simulink model "PI_MPC_PMSM"  (R2018b)
settings: Solver=ode23s  StartTime=0.0  StopTime=0.9  FixedStep=Ts  EnableMultiTasking=on
InitFcn:
  | Ts = 10e-6;
  | 
  | R = 0.958;
  | Ld = 5.25e-3;
  | Lq = 12e-3;
  | Pn = 4;
  | flux = 0.1827;
undefined symbols (not defined in the file): DiscIntNeverNeededParam
libraries: powerlib x7, powerlib_extras x3, simulink x2
settings Model: Creator=SUN  LastModifiedBy=Baize
settings SolverCC: ZeroCrossControl=DisableAll
settings DataIOCC: LimitDataPoints=on  SaveFormat=Array  SignalLoggingSaveFormat=ModelDataLogs
settings OptimizationCC: ExpressionDepthLimit=2147483647  InitFltsAndDblsToZero=on  LifeSpan=inf
settings DebuggingCC: UnderspecifiedInitializationDetection=Classic  MergeDetectMultiDrivingBlocksExec=none  SolverPrmCheckMsg=warning  FcnCallInpInsideContextMsg=warning  StateNameClashWarn=warning  SFUnexpectedBacktrackingDiag=warning  SFNoUnconditionalDefaultTransitionDiag=warning  SFExecutionAtInitializationDiag=none
settings HardwareCC: ProdBitPerPointer=32  ProdBitPerSizeT=32  ProdBitPerPtrDiffT=32  ProdLargestAtomicFloat=None  ProdIntDivRoundTo=Undefined  ProdEndianess=Unspecified  ProdWordSize=32  ProdHWDeviceType=32-bit Generic
settings ModelReferenceCC: PropagateSignalLabelsOutOfModel=off
settings SFSimCC: SimUseLocalCustomCode=off
settings RTWCC: RTWUseLocalCustomCode=off
settings CodeAppCC: StateflowObjectComments=on
settings GRTTargetCC: TargetLangStandard=C89/C90 (ANSI)  CombineOutputUpdateFcns=off  GRTInterface=on
settings ConfigComp: CovMetricSettings=dw  CovSaveCumulativeToWorkspaceVar=on  CovSaveSingleToWorkspaceVar=on  CovExternalEMLEnable=off  CovSFcnEnable=off
settings SimscapeCC: SimscapeNormalizeSystem=off

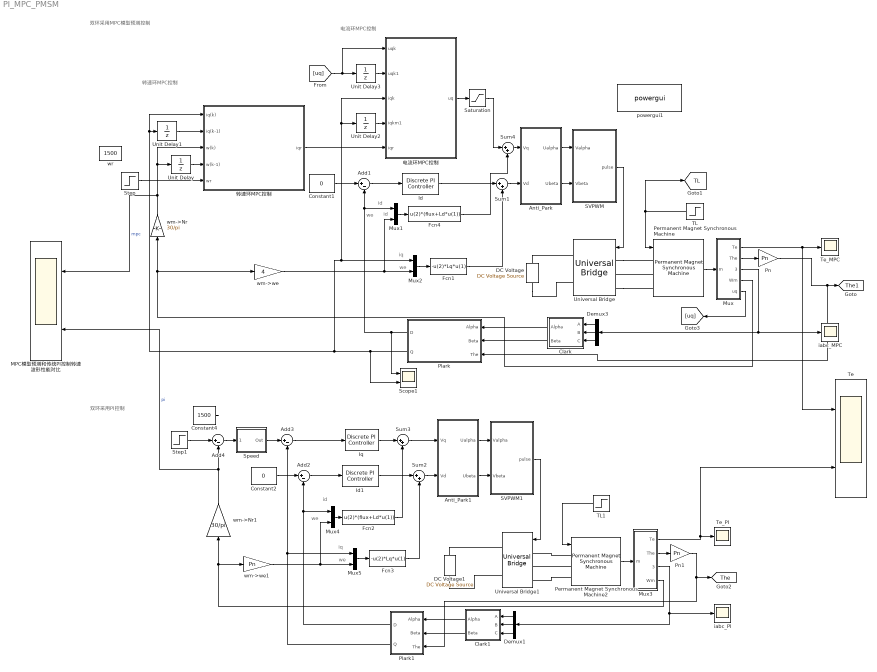
== system PI_MPC_PMSM ==
  note: 电流环MPC控制
  note: 转速环MPC控制
  note: 双环采用PI控制
  note: 双环采用MPC模型预测控制
  note: iq
  note: we
  note: id
  note: id
  note: iq
  note: we
  note: we
  note: we
  note: id
  Add{1..4} (4 alike) : Sum  Inputs=|+-
  Anti_Park : Subsystem
  Anti_Park1 : Subsystem
  Clark : Subsystem
  Clark1 : Subsystem
  Constant1 : Constant  Value=0
  Constant2 : Constant  Value=0
  Constant4 : Constant  Value=1500
  DC Voltage : powerlib/Electrical Sources/DC Voltage Source  Amplitude=540  Measurements=None
  DC Voltage1 : powerlib/Electrical Sources/DC Voltage Source  Amplitude=540  Measurements=None
  Demux1 : Demux  Outputs=3
  Demux3 : Demux  Outputs=3
  Fcn1 : Fcn  Expr=-u(2)*Lq*u(1)
  Fcn2 : Fcn  Expr=u(2)*(flux+Ld*u(1))
  Fcn3 : Fcn  Expr=-u(2)*Lq*u(1)
  Fcn4 : Fcn  Expr=u(2)*(flux+Ld*u(1))
  Id : powerlib_extras/Discrete  Control Blocks/Discrete PI Controller  Kp=Ld*1100  Ki=R*1100  Par_Limits=[311*0.9*sqrt(1/3) -311*0.9*sqrt(1/3)]  Init=0  Ts=Ts
  Id1 : powerlib_extras/Discrete  Control Blocks/Discrete PI Controller  Kp=Ld*1100  Ki=R*1100  Par_Limits=[311*0.9*sqrt(1/3) -311*0.9*sqrt(1/3)]  Init=0  Ts=Ts
  Iq : powerlib_extras/Discrete  Control Blocks/Discrete PI Controller  Kp=Lq*1100  Ki=R*1100  Par_Limits=[311*0.9*sqrt(1/3) -311*0.9*sqrt(1/3)]  Init=0  Ts=Ts
  MPC模型预测和传统PI控制转速波形性能对比 : Scope  NumInputPorts=2
  Mux : Subsystem
  Mux{1..2,4..5} (4 alike) : Mux  Inputs=2
  Mux3 : Subsystem
  Permanent Magnet Synchronous Machine : powerlib/Machines/Permanent Magnet Synchronous Machine  NbPhases=3  FluxDistribution=Sinusoidal  RotorType=Salient-pole  MechanicalLoad=Torque Tm  PresetModel=No  ShowDetailedParameters=on  MeasurementBus=off  Resistance=0.994  Inductance=8.5e-3  dqInductances=[6.3e-3,9e-3]  La=0.000395  MachineConstant=Flux linkage established by magnets (V.s)  Flux=0.3163  VoltageCst=229.4819  TorqueCst=1.8978  Flat=120  Mechanical=[0.014 0.009 4 0]  PolePairs=4  InitialConditions=[0,0,0,0]  InitialConditions5ph=[0 0 0 0 0 0]  TsPowergui=0  TsBlock=-1  RefAngle=Aligned with phase A axis (original Park)
      settings: SourceProductName=Simscape Power Systems
  Permanent Magnet Synchronous Machine2 : powerlib/Machines/Permanent Magnet Synchronous Machine  NbPhases=3  FluxDistribution=Sinusoidal  RotorType=Salient-pole  MechanicalLoad=Torque Tm  PresetModel=No  ShowDetailedParameters=on  MeasurementBus=off  Resistance=0.994  Inductance=8.5e-3  dqInductances=[6.3e-3,9e-3]  La=0.000395  MachineConstant=Flux linkage established by magnets (V.s)  Flux=0.3163  VoltageCst=229.4819  TorqueCst=1.8978  Flat=120  Mechanical=[0.014 0.009 4 0]  PolePairs=4  InitialConditions=[0,0,0,0]  InitialConditions5ph=[0 0 0 0 0 0]  TsPowergui=0  TsBlock=-1  RefAngle=Aligned with phase A axis (original Park)
      settings: SourceProductName=Simscape Power Systems
  Plark : Subsystem
  Plark1 : Subsystem
  Pn : Gain  Gain=Pn
  Pn1 : Gain  Gain=Pn
  SVPWM : Subsystem
  SVPWM1 : Subsystem
  Saturation : Saturate  UpperLimit=180  LowerLimit=-180
  Scope1 : Scope  NumInputPorts=2
  Speed : Subsystem  AncestorBlock=|  DialogController=POWERSYS.PowerSysDialog  mask(Discrete PI Controller){Kpw=0.14, Kiw=0.14*50, Ba=0.013, Par_Limits=[30 -30], Init=0, Ts=Ts}
      | powerlib_extras/Discrete 
      | Control Blocks/Discrete
      | PI Controller
      mask prompts: Kpw "Proportional gain (Kp):"; Kiw "Integral gain (Ki):"; Ba "feedback gain (Ba)"; Par_Limits "Output limits: [ Upper   Lower ]"; Init "Output initial value:"; Ts "Sample time:"
      mask help: This block implements a discrete PI controller.
      mask init:
      | UpperLimit=Par_Limits(1);
      | LowerLimit=Par_Limits(2);
      | power_initmask();
      mask Help: This block is part of a subset of blocks in the Extras library that does not have documentation associated with it, other than the block mask description.
      mask Display: disp('PI');
  Step : Step  Time=0.6  Before=1500  After=1300  SampleTime=0
  Step1 : Step  Time=0.6  Before=1500  After=1300  SampleTime=0
  Sum{1..4} (4 alike) : Sum  Inputs=|++
  TL : Step  Time=0.3  After=5  SampleTime=0
  TL1 : Step  Time=0.3  After=5  SampleTime=0
  Te : Scope  NumInputPorts=2
  Te_MPC : Scope
  Te_PI : Scope
  Unit Delay{,1..3} (4 alike) : UnitDelay  SampleTime=-1
  Universal Bridge : powerlib/Power Electronics/Universal Bridge  Arms=3  SnubberResistance=1e5  SnubberCapacitance=inf  Device=IGBT / Diodes  Ron=1e-3  Lon=0  ForwardVoltages="[  0  0  ]"  ForwardVoltage=0  GTOparameters=[ 10e-6 , 20e-6 ]  IGBTparameters=[ 1e-6 , 2e-6 ]  Measurements=None  Measurements_2=None  converterType=Rectifier
  Universal Bridge1 : powerlib/Power Electronics/Universal Bridge  Arms=3  SnubberResistance=1e5  SnubberCapacitance=inf  Device=IGBT / Diodes  Ron=1e-3  Lon=0  ForwardVoltages="[  0  0  ]"  ForwardVoltage=0  GTOparameters=[ 10e-6 , 20e-6 ]  IGBTparameters=[ 1e-6 , 2e-6 ]  Measurements=None  Measurements_2=None  converterType=Rectifier
  iabc_MPC : Scope
  iabc_PI : Scope
  powergui1 : powerlib/powergui  Priority=1  SimulationMode=Discrete  SampleTime=1e-6  frequency=60  Iterations=50  frequencyindice=0  Pbase=100e6  ErrMax=1e-4  UnitsV=kV  UnitsW=MW  buscounter=0  FunctionMessages=off  echomessages=off  EnableUseOfTLC=off  CurrentSourceSwitches=off  DisableSnubberDevices=off  DisableRonSwitches=off  DisableVfSwitches=off  DisplayEquations=off  SolverType=Tustin  Interpol=off  ExternalGateDelay=off  methode=off  Ts=10  x0status=blocks  SPID=off  SwTol=0  HookPort=off  RestoreLinks=warning  ResistiveCurrentMeasurement=off  Frange=[0:2:500]  Ylog=off  Xlog=on  ShowGrid=off  save=off  variable=ZData  structure=0  ZoomFFT=off  StartTime=0.0  cycles=1  DisplayStyle=1  fundamental=60  FreqAxis=off  MaxFrequency=1000  frequencyindicesteady=1  RmsSteady=1  display=off
  wm->Nr : Gain  Gain=30/pi
  wm->Nr1 : Gain  Gain=30/pi
  wm->we : Gain  Gain=4
  wm->we1 : Gain  Gain=Pn
  wr : Constant  Value=1500
  电流环MPC控制 : MATLAB Function  TreatAsAtomicUnit=on
  转速环MPC控制 : Subsystem
  tag scope: TL=global, The1=global, The=global
  wires:
  Permanent Magnet Synchronous Machine/1 -> Mux/1(m)
  Fcn1/1 -> Sum1/2
  Constant1/1 -> Add1/1
  Add1/1 -> Id/1
  wm->Nr/1 -> MPC模型预测和传统PI控制转速波形性能对比/1, 转速环MPC控制/3(w(k)), Unit Delay/1  "mpc"
  Id/1 -> Sum1/1
  Mux2/1 -> Fcn1/1
  Sum1/1 -> Anti_Park/2(Vd)
  Mux/1(Te) -> Te_MPC/1, Te/1
  Mux/2(The) -> Pn/1
  Pn/1 -> Plark/3(The), [The1]
  SVPWM/1(pulse) -> Universal Bridge/1
  Mux/4(Wm) -> wm->we/1, wm->Nr/1
  Mux/3(Iabc) -> iabc_MPC/1, Demux3/1
  Anti_Park/1(Ualpha) -> SVPWM/1(Valpha)
  Anti_Park/2(Ubeta) -> SVPWM/2(Vbeta)
  Clark/1(Alpha) -> Plark/1(Alpha)
  Demux3/1 -> Clark/1(A)
  Demux3/2 -> Clark/2(B)
  Demux3/3 -> Clark/3(C)
  Clark/2(Beta) -> Plark/2(Beta)
  TL/1 -> [TL], Permanent Magnet Synchronous Machine/1
  Unit Delay/1 -> 转速环MPC控制/4(w(k-1))
  Unit Delay1/1 -> 转速环MPC控制/2(iq(k-1))
  Step/1 -> 转速环MPC控制/5(wr)
  Add3/1 -> Iq/1
  Plark1/2(Q) -> Mux5/1, Add3/2
  Demux1/3 -> Clark1/3(C)
  SVPWM1/1(pulse) -> Universal Bridge1/1
  Mux3/2(The) -> Pn1/1
  Constant2/1 -> Add2/1
  Mux3/1(Te) -> Te/2, Te_PI/1
  Mux3/3(Iabc) -> iabc_PI/1, Demux1/1
  Sum2/1 -> Anti_Park1/2(Vd)
  Demux1/2 -> Clark1/2(B)
  Iq/1 -> Sum3/1
  Mux3/4(Wm) -> wm->we1/1, wm->Nr1/1
  Mux4/1 -> Fcn2/1
  Anti_Park1/2(Ubeta) -> SVPWM1/2(Vbeta)
  Add2/1 -> Id1/1
  wm->we1/1 -> Mux5/2, Mux4/2
  Constant4/1 -> ?
  Fcn3/1 -> Sum2/2
  Add4/1 -> Speed/1(Error)
  Permanent Magnet Synchronous Machine2/1 -> Mux3/1(m)
  Clark1/2(Beta) -> Plark1/2(Beta)
  wm->Nr1/1 -> Add4/2, MPC模型预测和传统PI控制转速波形性能对比/2  "pi"
  Demux1/1 -> Clark1/1(A)
  Speed/1(Out) -> Add3/1
  Mux5/1 -> Fcn3/1
  Id1/1 -> Sum2/1
  Clark1/1(Alpha) -> Plark1/1(Alpha)
  Plark1/1(D) -> Mux4/1, Add2/2
  Anti_Park1/1(Ualpha) -> SVPWM1/1(Valpha)
  Sum3/1 -> Anti_Park1/1(Vq)
  TL1/1 -> Permanent Magnet Synchronous Machine2/1
  Pn1/1 -> Plark1/3(The), [The]
  Fcn2/1 -> Sum3/2
  Plark/1(D) -> Scope1/1, Add1/2, Mux1/1
  Fcn4/1 -> Sum4/2
  Mux1/1 -> Fcn4/1
  wm->we/1 -> Mux2/2, Mux1/2
  Sum4/1 -> Anti_Park/1(Vq)
  Mux/5(uq) -> [uq]
  [uq] -> 电流环MPC控制/1(uqk), Unit Delay3/1
  Saturation/1 -> Sum4/1
  Unit Delay3/1 -> 电流环MPC控制/2(uqk1)
  电流环MPC控制/1(uq) -> Saturation/1
  Unit Delay2/1 -> 电流环MPC控制/4(iqkm1)
  转速环MPC控制/1(iqr) -> 电流环MPC控制/5(iqr)
  Plark/2(Q) -> Scope1/2, 转速环MPC控制/1(iq(k)), Unit Delay1/1, Mux2/1, 电流环MPC控制/3(iqk), Unit Delay2/1
  Step1/1 -> Add4/1
  connections:
  Permanent Magnet Synchronous Machine/LConn2 -- Universal Bridge/LConn2
  DC Voltage/RConn1 -- Universal Bridge/RConn1
  DC Voltage/LConn1 -- Universal Bridge/RConn2
  Universal Bridge/LConn3 -- Permanent Magnet Synchronous Machine/LConn3
  Universal Bridge/LConn1 -- Permanent Magnet Synchronous Machine/LConn1
  Permanent Magnet Synchronous Machine2/LConn2 -- Universal Bridge1/LConn2
  Permanent Magnet Synchronous Machine2/LConn1 -- Universal Bridge1/LConn1
  Permanent Magnet Synchronous Machine2/LConn3 -- Universal Bridge1/LConn3
  DC Voltage1/RConn1 -- Universal Bridge1/RConn1
  DC Voltage1/LConn1 -- Universal Bridge1/RConn2

== system PI_MPC_PMSM/Anti_Park ==
  Vq : Inport
  Vd : Inport  Port=2
  Fcn : Fcn  Expr=cos(u[1])*u[2]-sin(u[1])*u[3]
  Fcn1 : Fcn  Expr=sin(u[1])*u[2]+cos(u[1])*u[3]
  Mux1 : Mux  Inputs=3
  Ualpha : Outport  VectorParamsAs1DForOutWhenUnconnected=on
  Ubeta : Outport  Port=2  VectorParamsAs1DForOutWhenUnconnected=on
  wires:
  Fcn1/1 -> Ubeta/1
  Fcn/1 -> Ualpha/1
  Mux1/1 -> Fcn/1, Fcn1/1
  Vd/1 -> Mux1/2
  Vq/1 -> Mux1/3
  [The1] -> Mux1/1

== system PI_MPC_PMSM/Anti_Park1 ==
  Vq : Inport
  Vd : Inport  Port=2
  Fcn : Fcn  Expr=cos(u[1])*u[2]-sin(u[1])*u[3]
  Fcn1 : Fcn  Expr=sin(u[1])*u[2]+cos(u[1])*u[3]
  Mux1 : Mux  Inputs=3
  Ualpha : Outport  VectorParamsAs1DForOutWhenUnconnected=on
  Ubeta : Outport  Port=2  VectorParamsAs1DForOutWhenUnconnected=on
  wires:
  Fcn1/1 -> Ubeta/1
  Fcn/1 -> Ualpha/1
  Mux1/1 -> Fcn/1, Fcn1/1
  Vd/1 -> Mux1/2
  Vq/1 -> Mux1/3
  [The] -> Mux1/1

== system PI_MPC_PMSM/Clark ==
  A : Inport
  B : Inport  Port=2
  C : Inport  Port=3
  Mux : Mux  Inputs=3
  alpha : Fcn  Expr=(u(1)-0.5*(u(2)+u(3)))*2/3
  beta : Fcn  Expr=sqrt(3)/2*(u(2)-u(3))*2/3
  Alpha : Outport  VectorParamsAs1DForOutWhenUnconnected=on
  Beta : Outport  Port=2  VectorParamsAs1DForOutWhenUnconnected=on
  wires:
  alpha/1 -> Alpha/1
  B/1 -> Mux/2
  C/1 -> Mux/3
  A/1 -> Mux/1
  Mux/1 -> beta/1, alpha/1
  beta/1 -> Beta/1

== system PI_MPC_PMSM/Clark1 ==
  A : Inport
  B : Inport  Port=2
  C : Inport  Port=3
  Mux : Mux  Inputs=3
  alpha : Fcn  Expr=(u(1)-0.5*(u(2)+u(3)))*2/3
  beta : Fcn  Expr=sqrt(3)/2*(u(2)-u(3))*2/3
  Alpha : Outport  VectorParamsAs1DForOutWhenUnconnected=on
  Beta : Outport  Port=2  VectorParamsAs1DForOutWhenUnconnected=on
  wires:
  alpha/1 -> Alpha/1
  B/1 -> Mux/2
  C/1 -> Mux/3
  A/1 -> Mux/1
  Mux/1 -> beta/1, alpha/1
  beta/1 -> Beta/1

== system PI_MPC_PMSM/Mux ==
  m : Inport
  Bus Selector : BusSelector  OutputSignals=Stator current is_a (A),Stator current is_b (A),Stator current is_c (A)
  Bus Selector1 : BusSelector  OutputSignals=Rotor speed wm (rad/s),Rotor angle thetam (rad),Electromagnetic torque Te (N*m),Stator voltage Vs_q (V)
  Mux : Mux  Inputs=3
  Te : Outport  VectorParamsAs1DForOutWhenUnconnected=on
  The : Outport  Port=2  VectorParamsAs1DForOutWhenUnconnected=on
  Iabc : Outport  Port=3  VectorParamsAs1DForOutWhenUnconnected=on
  Wm : Outport  Port=4  VectorParamsAs1DForOutWhenUnconnected=on
  uq : Outport  Port=5  VectorParamsAs1DForOutWhenUnconnected=on
  wires:
  Bus Selector1/1 -> Wm/1  "<Rotor speed wm (rad/s)>"
  Bus Selector1/2 -> The/1  "<Rotor angle thetam (rad)>"
  Bus Selector1/3 -> Te/1  "<Electromagnetic torque Te (N*m)>"
  m/1 -> Bus Selector/1, Bus Selector1/1
  Bus Selector/2 -> Mux/2  "<Stator current is_b (A)>"
  Bus Selector/3 -> Mux/3  "<Stator current is_c (A)>"
  Bus Selector/1 -> Mux/1  "<Stator current is_a (A)>"
  Mux/1 -> Iabc/1
  Bus Selector1/4 -> uq/1  "<Stator voltage Vs_q (V)>"

== system PI_MPC_PMSM/Mux3 ==
  m : Inport
  Bus Selector : BusSelector  OutputSignals=Stator current is_a (A),Stator current is_b (A),Stator current is_c (A)
  Bus Selector1 : BusSelector  OutputSignals=Rotor speed wm (rad/s),Rotor angle thetam (rad),Electromagnetic torque Te (N*m)
  Mux : Mux  Inputs=3
  Te : Outport  VectorParamsAs1DForOutWhenUnconnected=on
  The : Outport  Port=2  VectorParamsAs1DForOutWhenUnconnected=on
  Iabc : Outport  Port=3  VectorParamsAs1DForOutWhenUnconnected=on
  Wm : Outport  Port=4  VectorParamsAs1DForOutWhenUnconnected=on
  wires:
  Bus Selector1/1 -> Wm/1  "<Rotor speed wm (rad/s)>"
  Bus Selector1/2 -> The/1  "<Rotor angle thetam (rad)>"
  Bus Selector1/3 -> Te/1  "<Electromagnetic torque Te (N*m)>"
  m/1 -> Bus Selector/1, Bus Selector1/1
  Bus Selector/2 -> Mux/2  "<Stator current is_b (A)>"
  Bus Selector/3 -> Mux/3  "<Stator current is_c (A)>"
  Bus Selector/1 -> Mux/1  "<Stator current is_a (A)>"
  Mux/1 -> Iabc/1

== system PI_MPC_PMSM/Plark ==
  Alpha : Inport
  Beta : Inport  Port=2
  The : Inport  Port=3
  Mux : Mux  Inputs=3
  d : Fcn  Expr=u(1)*cos(u(3))+u(2)*sin(u(3))
  q : Fcn  Expr=-u(1)*sin(u(3))+u(2)*cos(u(3))
  D : Outport  VectorParamsAs1DForOutWhenUnconnected=on
  Q : Outport  Port=2  VectorParamsAs1DForOutWhenUnconnected=on
  wires:
  d/1 -> D/1
  Beta/1 -> Mux/2
  Alpha/1 -> Mux/1
  Mux/1 -> q/1, d/1
  q/1 -> Q/1
  The/1 -> Mux/3

== system PI_MPC_PMSM/Plark1 ==
  Alpha : Inport
  Beta : Inport  Port=2
  The : Inport  Port=3
  Mux : Mux  Inputs=3
  d : Fcn  Expr=u(1)*cos(u(3))+u(2)*sin(u(3))
  q : Fcn  Expr=-u(1)*sin(u(3))+u(2)*cos(u(3))
  D : Outport  VectorParamsAs1DForOutWhenUnconnected=on
  Q : Outport  Port=2  VectorParamsAs1DForOutWhenUnconnected=on
  wires:
  d/1 -> D/1
  Beta/1 -> Mux/2
  Alpha/1 -> Mux/1
  Mux/1 -> q/1, d/1
  q/1 -> Q/1
  The/1 -> Mux/3

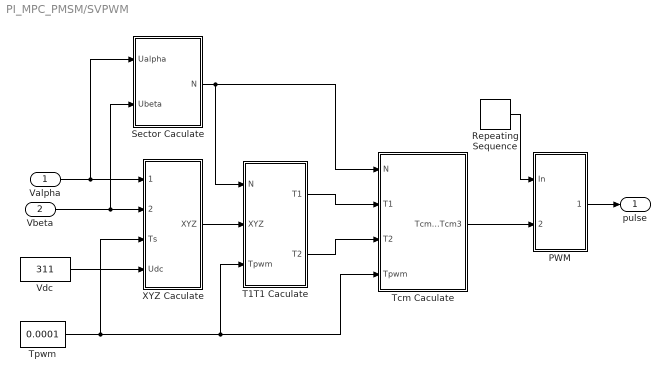
== system PI_MPC_PMSM/SVPWM ==
  Valpha : Inport
  Vbeta : Inport  Port=2
  PWM : Subsystem
  Repeating Sequence : simulink/Sources/Repeating Sequence  rep_seq_t=[0 0.00005 0.0001]  rep_seq_y=[0 0.00005 0]
  Sector Caculate : Subsystem
  T1T1 Caculate : Subsystem
  Tcm Caculate : Subsystem
  Tpwm : Constant  Value=0.0001
  Vdc : Constant  Value=311
  XYZ Caculate : Subsystem
  pulse : Outport  VectorParamsAs1DForOutWhenUnconnected=on
  wires:
  PWM/1(PWM) -> pulse/1
  Repeating Sequence/1 -> PWM/1(In)
  Vbeta/1 -> XYZ Caculate/2(Ubeta), Sector Caculate/2(Ubeta)
  T1T1 Caculate/1(T1) -> Tcm Caculate/2(T1)
  Valpha/1 -> XYZ Caculate/1(Ualpha), Sector Caculate/1(Ualpha)
  T1T1 Caculate/2(T2) -> Tcm Caculate/3(T2)
  Sector Caculate/1("N ") -> Tcm Caculate/1(N), T1T1 Caculate/1(N)
  XYZ Caculate/1(XYZ) -> T1T1 Caculate/2(XYZ)
  Tpwm/1 -> XYZ Caculate/3(Ts), Tcm Caculate/4(Tpwm), T1T1 Caculate/3(Tpwm)
  Vdc/1 -> XYZ Caculate/4(Udc)
  Tcm Caculate/1(Tcm1 Tcm2 Tcm3) -> PWM/2(Tcm123)

== system PI_MPC_PMSM/SVPWM1 ==
  Valpha : Inport
  Vbeta : Inport  Port=2
  PWM : Subsystem
  Repeating Sequence : simulink/Sources/Repeating Sequence  rep_seq_t=[0 0.00005 0.0001]  rep_seq_y=[0 0.00005 0]
  Sector Caculate : Subsystem
  T1T1 Caculate : Subsystem
  Tcm Caculate : Subsystem
  Tpwm : Constant  Value=0.0001
  Vdc : Constant  Value=311
  XYZ Caculate : Subsystem
  pulse : Outport  VectorParamsAs1DForOutWhenUnconnected=on
  wires:
  PWM/1(PWM) -> pulse/1
  Repeating Sequence/1 -> PWM/1(In)
  Vbeta/1 -> XYZ Caculate/2(Ubeta), Sector Caculate/2(Ubeta)
  T1T1 Caculate/1(T1) -> Tcm Caculate/2(T1)
  Valpha/1 -> XYZ Caculate/1(Ualpha), Sector Caculate/1(Ualpha)
  T1T1 Caculate/2(T2) -> Tcm Caculate/3(T2)
  Sector Caculate/1("N ") -> Tcm Caculate/1(N), T1T1 Caculate/1(N)
  XYZ Caculate/1(XYZ) -> T1T1 Caculate/2(XYZ)
  Tpwm/1 -> XYZ Caculate/3(Ts), Tcm Caculate/4(Tpwm), T1T1 Caculate/3(Tpwm)
  Vdc/1 -> XYZ Caculate/4(Udc)
  Tcm Caculate/1(Tcm1 Tcm2 Tcm3) -> PWM/2(Tcm123)

== system PI_MPC_PMSM/Speed ==
  note: Discrete PID Controller
  Error : Inport  SampleTime=Ts
  Discrete-Time Integrator : DiscreteIntegrator  InitialCondition=Init  SampleTime=Ts  LimitOutput=on  UpperSaturationLimit=UpperLimit  LowerSaturationLimit=LowerLimit  ICPrevOutput=DiscIntNeverNeededParam  ICPrevScaledInput=DiscIntNeverNeededParam
  Kp1 : Gain  Gain=Ba  SampleTime=Ts  SaturateOnIntegerOverflow=on  OutDataTypeStr=Inherit: Same as input  ParamDataTypeStr=Inherit: Same as input
  Kp4 : Gain  Gain=Kpw  SampleTime=Ts  SaturateOnIntegerOverflow=on  OutDataTypeStr=Inherit: Same as input  ParamDataTypeStr=Inherit: Same as input
  Kp5 : Gain  Gain=Kiw  SampleTime=Ts  SaturateOnIntegerOverflow=on  OutDataTypeStr=Inherit: Same as input  ParamDataTypeStr=Inherit: Same as input
  Saturation2 : Saturate  UpperLimit=UpperLimit  LowerLimit=LowerLimit  SampleTime=Ts
  Sum6 : Sum  Inputs=++-  SampleTime=Ts  SaturateOnIntegerOverflow=on  InputSameDT=on  OutDataTypeStr=Inherit: Same as first input
  Zero-Order Hold : ZeroOrderHold  SampleTime=Ts
  Out : Outport  SampleTime=Ts  InitialOutput=0  VectorParamsAs1DForOutWhenUnconnected=on
  wires:
  Error/1 -> Kp1/1, Kp5/1, Kp4/1
  Zero-Order Hold/1 -> Sum6/1
  Saturation2/1 -> Out/1
  Discrete-Time Integrator/1 -> Sum6/2
  Kp4/1 -> Zero-Order Hold/1
  Kp5/1 -> Discrete-Time Integrator/1
  Sum6/1 -> Saturation2/1
  Kp1/1 -> Sum6/3

== system PI_MPC_PMSM/转速环MPC控制 ==
  iq(k) : Inport
  iq(k-1) : Inport  Port=2
  w(k) : Inport  Port=3
  w(k-1) : Inport  Port=4
  wr : Inport  Port=5
  MATLAB Function : MATLAB Function  TreatAsAtomicUnit=on
  Saturation : Saturate  UpperLimit=30  LowerLimit=-30
  iqr : Outport  VectorParamsAs1DForOutWhenUnconnected=on
  wires:
  w(k-1)/1 -> MATLAB Function/4(wk1)
  iq(k-1)/1 -> MATLAB Function/2(iqk1)
  iq(k)/1 -> MATLAB Function/1(iqk)
  MATLAB Function/1(iq) -> Saturation/1
  w(k)/1 -> MATLAB Function/3(wk)
  wr/1 -> MATLAB Function/5(wr)
  Saturation/1 -> iqr/1
  [TL] -> MATLAB Function/6(TL)

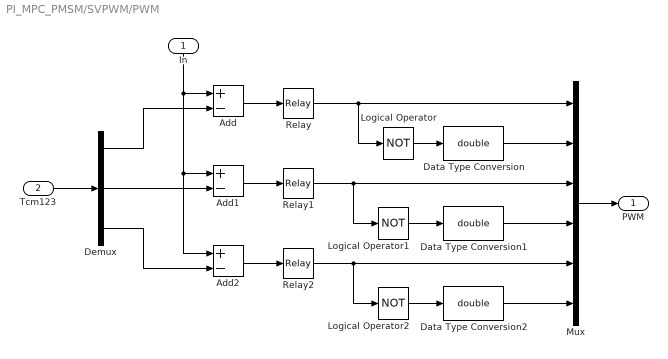
== system PI_MPC_PMSM/SVPWM/PWM ==
  In : Inport
  Tcm123 : Inport  Port=2
  Add : Sum  Inputs=+-
  Add1 : Sum  Inputs=+-
  Add2 : Sum  Inputs=+-
  Data Type Conversion : DataTypeConversion  OutDataTypeStr=double
  Data Type Conversion1 : DataTypeConversion  OutDataTypeStr=double
  Data Type Conversion2 : DataTypeConversion  OutDataTypeStr=double
  Demux : Demux  Outputs=3
  Logical Operator : Logic  Operator=NOT  AllPortsSameDT=off  OutDataTypeStr=boolean
  Logical Operator1 : Logic  Operator=NOT  AllPortsSameDT=off  OutDataTypeStr=boolean
  Logical Operator2 : Logic  Operator=NOT  AllPortsSameDT=off  OutDataTypeStr=boolean
  Mux : Mux  Inputs=6
  Relay : Relay  OffSwitchValue=-eps
  Relay1 : Relay  OffSwitchValue=-eps
  Relay2 : Relay  OffSwitchValue=-eps
  PWM : Outport  VectorParamsAs1DForOutWhenUnconnected=on
  wires:
  Demux/3 -> Add2/2
  Demux/2 -> Add1/2
  Demux/1 -> Add/2
  Relay2/1 -> Mux/5, Logical Operator2/1
  Relay1/1 -> Mux/3, Logical Operator1/1
  Relay/1 -> Logical Operator/1, Mux/1
  Mux/1 -> PWM/1
  Data Type Conversion/1 -> Mux/2
  Data Type Conversion1/1 -> Mux/4
  Data Type Conversion2/1 -> Mux/6
  Logical Operator2/1 -> Data Type Conversion2/1
  Logical Operator1/1 -> Data Type Conversion1/1
  Logical Operator/1 -> Data Type Conversion/1
  Add1/1 -> Relay1/1
  Add2/1 -> Relay2/1
  Add/1 -> Relay/1
  In/1 -> Add/1, Add2/1, Add1/1
  Tcm123/1 -> Demux/1

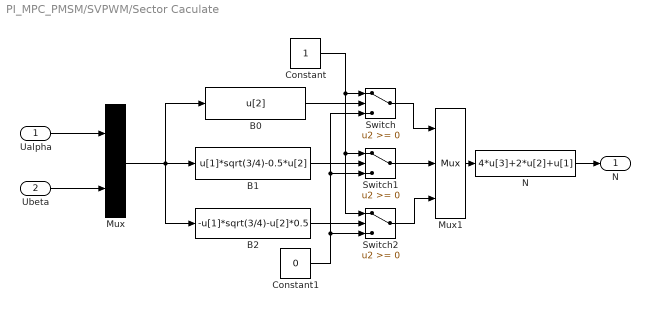
== system PI_MPC_PMSM/SVPWM/Sector Caculate ==
  Ualpha : Inport
  Ubeta : Inport  Port=2
  B0 : Fcn  Expr=u[2]
  B1 : Fcn  Expr=u[1]*sqrt(3/4)-0.5*u[2]
  B2 : Fcn  Expr=-u[1]*sqrt(3/4)-u[2]*0.5
  Constant : Constant
  Constant1 : Constant  Value=0
  Mux : Mux  Inputs=2
  Mux1 : Mux  Inputs=3
  N : Fcn  Expr=4*u[3]+2*u[2]+u[1]
  Switch : Switch
  Switch1 : Switch
  Switch2 : Switch
  "N " : Outport  VectorParamsAs1DForOutWhenUnconnected=on
  wires:
  Switch2/1 -> Mux1/3
  Switch/1 -> Mux1/1
  Ualpha/1 -> Mux/1
  Ubeta/1 -> Mux/2
  Mux/1 -> B2/1, B1/1, B0/1
  B0/1 -> Switch/2
  B1/1 -> Switch1/2
  B2/1 -> Switch2/2
  Constant/1 -> Switch/1, Switch2/1, Switch1/1
  Constant1/1 -> Switch/3, Switch1/3, Switch2/3
  Switch1/1 -> Mux1/2
  Mux1/1 -> N/1
  N/1 -> "N "/1

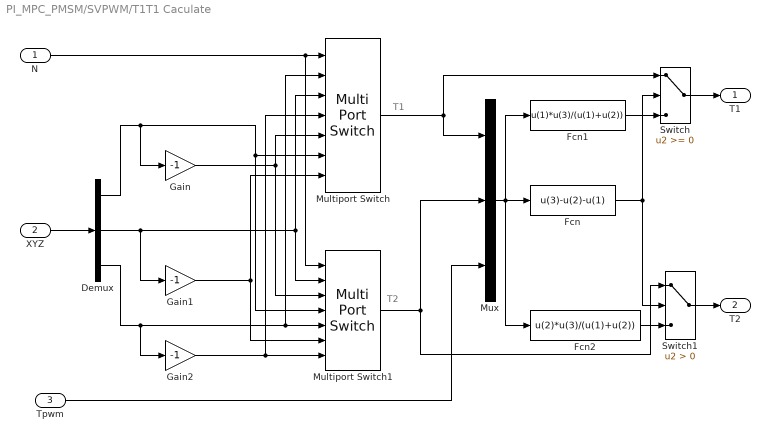
== system PI_MPC_PMSM/SVPWM/T1T1 Caculate ==
  note: T1
  note: T2
  N : Inport
  XYZ : Inport  Port=2
  Tpwm : Inport  Port=3
  Demux : Demux  Outputs=3
  Fcn : Fcn  Expr=u(3)-u(2)-u(1)
  Fcn1 : Fcn  Expr=u(1)*u(3)/(u(1)+u(2))
  Fcn2 : Fcn  Expr=u(2)*u(3)/(u(1)+u(2))
  Gain : Gain  Gain=-1
  Gain1 : Gain  Gain=-1
  Gain2 : Gain  Gain=-1
  Multiport Switch : MultiPortSwitch  Inputs=6
  Multiport Switch1 : MultiPortSwitch  Inputs=6
  Mux : Mux  Inputs=3
  Switch : Switch
  Switch1 : Switch  Criteria=u2 > Threshold
  T1 : Outport  VectorParamsAs1DForOutWhenUnconnected=on
  T2 : Outport  Port=2  VectorParamsAs1DForOutWhenUnconnected=on
  wires:
  Tpwm/1 -> Mux/3
  XYZ/1 -> Demux/1
  Switch1/1 -> T2/1
  Switch/1 -> T1/1
  Fcn2/1 -> Switch1/3
  Fcn1/1 -> Switch/3
  Fcn/1 -> Switch/2, Switch1/2
  Mux/1 -> Fcn1/1, Fcn/1, Fcn2/1
  Multiport Switch/1 -> Switch/1, Mux/1
  Multiport Switch1/1 -> Switch1/1, Mux/2
  N/1 -> Multiport Switch/1, Multiport Switch1/1
  Demux/2 -> Multiport Switch/3, Multiport Switch1/2, Gain1/1
  Demux/3 -> Multiport Switch1/5, Multiport Switch/2, Gain2/1
  Demux/1 -> Multiport Switch/6, Multiport Switch1/4, Gain/1
  Gain/1 -> Multiport Switch1/3, Multiport Switch/5
  Gain2/1 -> Multiport Switch/4, Multiport Switch1/7
  Gain1/1 -> Multiport Switch1/6, Multiport Switch/7

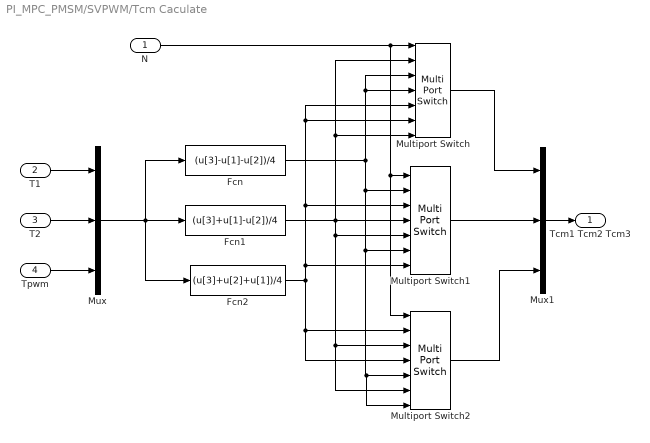
== system PI_MPC_PMSM/SVPWM/Tcm Caculate ==
  N : Inport
  T1 : Inport  Port=2
  T2 : Inport  Port=3
  Tpwm : Inport  Port=4
  Fcn : Fcn  Expr=(u[3]-u[1]-u[2])/4
  Fcn1 : Fcn  Expr=(u[3]+u[1]-u[2])/4
  Fcn2 : Fcn  Expr=(u[3]+u[2]+u[1])/4
  Multiport Switch : MultiPortSwitch  Inputs=6
  Multiport Switch1 : MultiPortSwitch  Inputs=6
  Multiport Switch2 : MultiPortSwitch  Inputs=6
  Mux : Mux  Inputs=3
  Mux1 : Mux  Inputs=3
  Tcm1 Tcm2 Tcm3 : Outport  VectorParamsAs1DForOutWhenUnconnected=on
  wires:
  Mux/1 -> Fcn2/1, Fcn/1, Fcn1/1
  Tpwm/1 -> Mux/3
  T2/1 -> Mux/2
  T1/1 -> Mux/1
  Multiport Switch2/1 -> Mux1/3
  Multiport Switch1/1 -> Mux1/2
  Multiport Switch/1 -> Mux1/1
  Mux1/1 -> Tcm1 Tcm2 Tcm3/1
  Fcn/1 -> Multiport Switch/3, Multiport Switch/4, Multiport Switch1/6, Multiport Switch2/5, Multiport Switch2/7, Multiport Switch1/2
  Fcn1/1 -> Multiport Switch1/5, Multiport Switch2/3, Multiport Switch2/6, Multiport Switch1/4, Multiport Switch/7, Multiport Switch/2
  Fcn2/1 -> Multiport Switch/5, Multiport Switch/6, Multiport Switch1/3, Multiport Switch1/7, Multiport Switch2/2, Multiport Switch2/4
  N/1 -> Multiport Switch2/1, Multiport Switch1/1, Multiport Switch/1

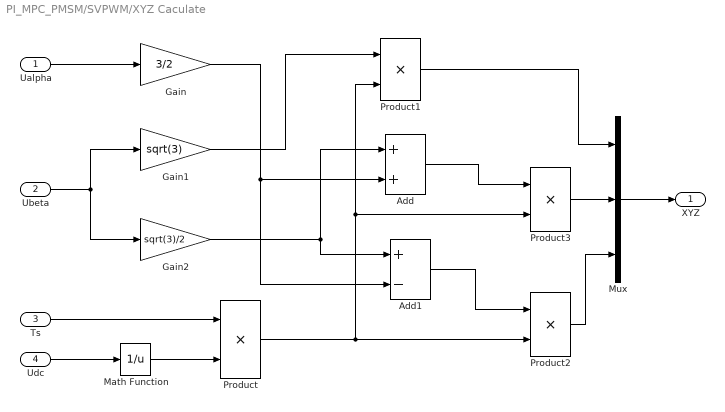
== system PI_MPC_PMSM/SVPWM/XYZ Caculate ==
  Ualpha : Inport
  Ubeta : Inport  Port=2
  Ts : Inport  Port=3
  Udc : Inport  Port=4
  Add : Sum
  Add1 : Sum  Inputs=+-
  Gain : Gain  Gain=3/2
  Gain1 : Gain  Gain=sqrt(3)
  Gain2 : Gain  Gain=sqrt(3)/2
  Math Function : Math  Operator=reciprocal  SaturateOnIntegerOverflow=on
  Mux : Mux  Inputs=3
  Product{,1..3} (4 alike) : Product  RndMeth=Zero
  XYZ : Outport  VectorParamsAs1DForOutWhenUnconnected=on
  wires:
  Mux/1 -> XYZ/1
  Product1/1 -> Mux/1
  Product3/1 -> Mux/2
  Product2/1 -> Mux/3
  Ualpha/1 -> Gain/1
  Ubeta/1 -> Gain2/1, Gain1/1
  Udc/1 -> Math Function/1
  Math Function/1 -> Product/2
  Ts/1 -> Product/1
  Gain1/1 -> Product1/1
  Product/1 -> Product2/2, Product1/2, Product3/2
  Gain/1 -> Add1/2, Add/2
  Gain2/1 -> Add/1, Add1/1
  Add1/1 -> Product2/1
  Add/1 -> Product3/1

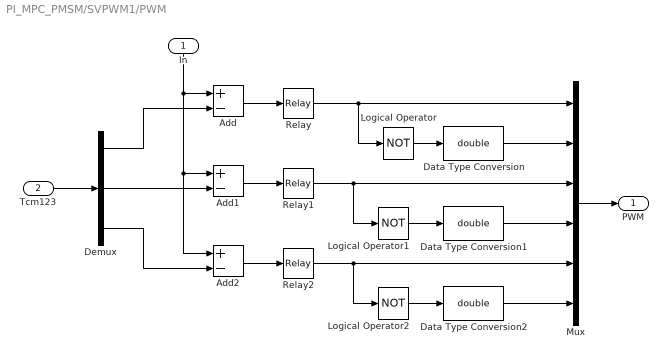
== system PI_MPC_PMSM/SVPWM1/PWM ==
  In : Inport
  Tcm123 : Inport  Port=2
  Add : Sum  Inputs=+-
  Add1 : Sum  Inputs=+-
  Add2 : Sum  Inputs=+-
  Data Type Conversion : DataTypeConversion  OutDataTypeStr=double
  Data Type Conversion1 : DataTypeConversion  OutDataTypeStr=double
  Data Type Conversion2 : DataTypeConversion  OutDataTypeStr=double
  Demux : Demux  Outputs=3
  Logical Operator : Logic  Operator=NOT  AllPortsSameDT=off  OutDataTypeStr=boolean
  Logical Operator1 : Logic  Operator=NOT  AllPortsSameDT=off  OutDataTypeStr=boolean
  Logical Operator2 : Logic  Operator=NOT  AllPortsSameDT=off  OutDataTypeStr=boolean
  Mux : Mux  Inputs=6
  Relay : Relay  OffSwitchValue=-eps
  Relay1 : Relay  OffSwitchValue=-eps
  Relay2 : Relay  OffSwitchValue=-eps
  PWM : Outport  VectorParamsAs1DForOutWhenUnconnected=on
  wires:
  Demux/3 -> Add2/2
  Demux/2 -> Add1/2
  Demux/1 -> Add/2
  Relay2/1 -> Mux/5, Logical Operator2/1
  Relay1/1 -> Mux/3, Logical Operator1/1
  Relay/1 -> Logical Operator/1, Mux/1
  Mux/1 -> PWM/1
  Data Type Conversion/1 -> Mux/2
  Data Type Conversion1/1 -> Mux/4
  Data Type Conversion2/1 -> Mux/6
  Logical Operator2/1 -> Data Type Conversion2/1
  Logical Operator1/1 -> Data Type Conversion1/1
  Logical Operator/1 -> Data Type Conversion/1
  Add1/1 -> Relay1/1
  Add2/1 -> Relay2/1
  Add/1 -> Relay/1
  In/1 -> Add/1, Add2/1, Add1/1
  Tcm123/1 -> Demux/1

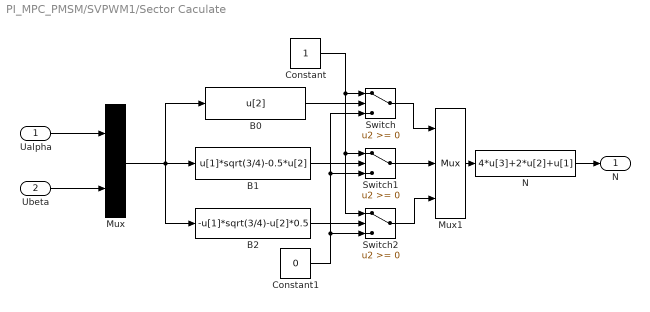
== system PI_MPC_PMSM/SVPWM1/Sector Caculate ==
  Ualpha : Inport
  Ubeta : Inport  Port=2
  B0 : Fcn  Expr=u[2]
  B1 : Fcn  Expr=u[1]*sqrt(3/4)-0.5*u[2]
  B2 : Fcn  Expr=-u[1]*sqrt(3/4)-u[2]*0.5
  Constant : Constant
  Constant1 : Constant  Value=0
  Mux : Mux  Inputs=2
  Mux1 : Mux  Inputs=3
  N : Fcn  Expr=4*u[3]+2*u[2]+u[1]
  Switch : Switch
  Switch1 : Switch
  Switch2 : Switch
  "N " : Outport  VectorParamsAs1DForOutWhenUnconnected=on
  wires:
  Switch2/1 -> Mux1/3
  Switch/1 -> Mux1/1
  Ualpha/1 -> Mux/1
  Ubeta/1 -> Mux/2
  Mux/1 -> B2/1, B1/1, B0/1
  B0/1 -> Switch/2
  B1/1 -> Switch1/2
  B2/1 -> Switch2/2
  Constant/1 -> Switch/1, Switch2/1, Switch1/1
  Constant1/1 -> Switch/3, Switch1/3, Switch2/3
  Switch1/1 -> Mux1/2
  Mux1/1 -> N/1
  N/1 -> "N "/1

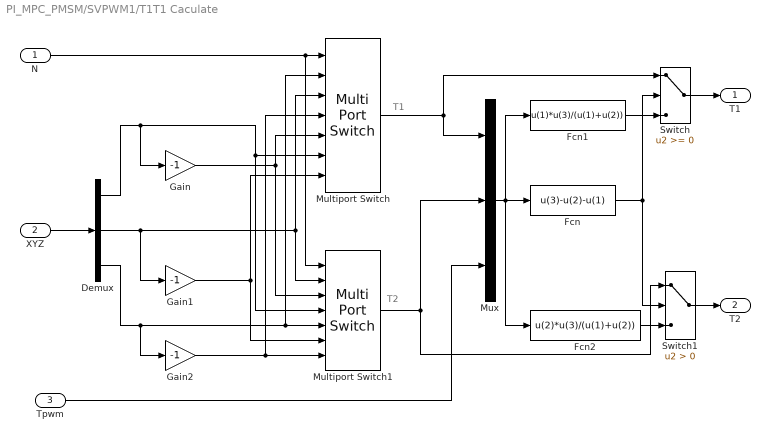
== system PI_MPC_PMSM/SVPWM1/T1T1 Caculate ==
  note: T1
  note: T2
  N : Inport
  XYZ : Inport  Port=2
  Tpwm : Inport  Port=3
  Demux : Demux  Outputs=3
  Fcn : Fcn  Expr=u(3)-u(2)-u(1)
  Fcn1 : Fcn  Expr=u(1)*u(3)/(u(1)+u(2))
  Fcn2 : Fcn  Expr=u(2)*u(3)/(u(1)+u(2))
  Gain : Gain  Gain=-1
  Gain1 : Gain  Gain=-1
  Gain2 : Gain  Gain=-1
  Multiport Switch : MultiPortSwitch  Inputs=6
  Multiport Switch1 : MultiPortSwitch  Inputs=6
  Mux : Mux  Inputs=3
  Switch : Switch
  Switch1 : Switch  Criteria=u2 > Threshold
  T1 : Outport  VectorParamsAs1DForOutWhenUnconnected=on
  T2 : Outport  Port=2  VectorParamsAs1DForOutWhenUnconnected=on
  wires:
  Tpwm/1 -> Mux/3
  XYZ/1 -> Demux/1
  Switch1/1 -> T2/1
  Switch/1 -> T1/1
  Fcn2/1 -> Switch1/3
  Fcn1/1 -> Switch/3
  Fcn/1 -> Switch/2, Switch1/2
  Mux/1 -> Fcn1/1, Fcn/1, Fcn2/1
  Multiport Switch/1 -> Switch/1, Mux/1
  Multiport Switch1/1 -> Switch1/1, Mux/2
  N/1 -> Multiport Switch/1, Multiport Switch1/1
  Demux/2 -> Multiport Switch/3, Multiport Switch1/2, Gain1/1
  Demux/3 -> Multiport Switch1/5, Multiport Switch/2, Gain2/1
  Demux/1 -> Multiport Switch/6, Multiport Switch1/4, Gain/1
  Gain/1 -> Multiport Switch1/3, Multiport Switch/5
  Gain2/1 -> Multiport Switch/4, Multiport Switch1/7
  Gain1/1 -> Multiport Switch1/6, Multiport Switch/7

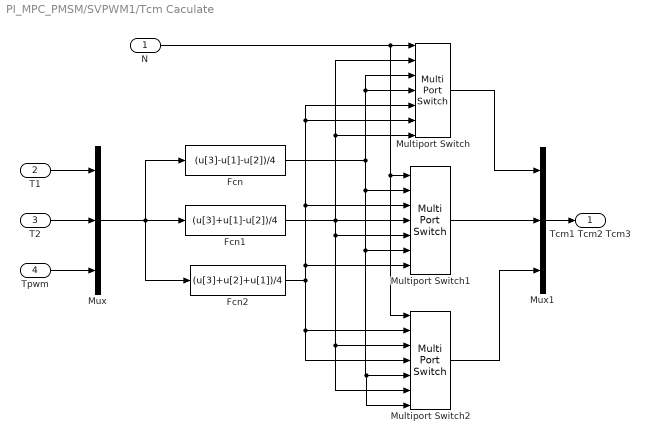
== system PI_MPC_PMSM/SVPWM1/Tcm Caculate ==
  N : Inport
  T1 : Inport  Port=2
  T2 : Inport  Port=3
  Tpwm : Inport  Port=4
  Fcn : Fcn  Expr=(u[3]-u[1]-u[2])/4
  Fcn1 : Fcn  Expr=(u[3]+u[1]-u[2])/4
  Fcn2 : Fcn  Expr=(u[3]+u[2]+u[1])/4
  Multiport Switch : MultiPortSwitch  Inputs=6
  Multiport Switch1 : MultiPortSwitch  Inputs=6
  Multiport Switch2 : MultiPortSwitch  Inputs=6
  Mux : Mux  Inputs=3
  Mux1 : Mux  Inputs=3
  Tcm1 Tcm2 Tcm3 : Outport  VectorParamsAs1DForOutWhenUnconnected=on
  wires:
  Mux/1 -> Fcn2/1, Fcn/1, Fcn1/1
  Tpwm/1 -> Mux/3
  T2/1 -> Mux/2
  T1/1 -> Mux/1
  Multiport Switch2/1 -> Mux1/3
  Multiport Switch1/1 -> Mux1/2
  Multiport Switch/1 -> Mux1/1
  Mux1/1 -> Tcm1 Tcm2 Tcm3/1
  Fcn/1 -> Multiport Switch/3, Multiport Switch/4, Multiport Switch1/6, Multiport Switch2/5, Multiport Switch2/7, Multiport Switch1/2
  Fcn1/1 -> Multiport Switch1/5, Multiport Switch2/3, Multiport Switch2/6, Multiport Switch1/4, Multiport Switch/7, Multiport Switch/2
  Fcn2/1 -> Multiport Switch/5, Multiport Switch/6, Multiport Switch1/3, Multiport Switch1/7, Multiport Switch2/2, Multiport Switch2/4
  N/1 -> Multiport Switch2/1, Multiport Switch1/1, Multiport Switch/1

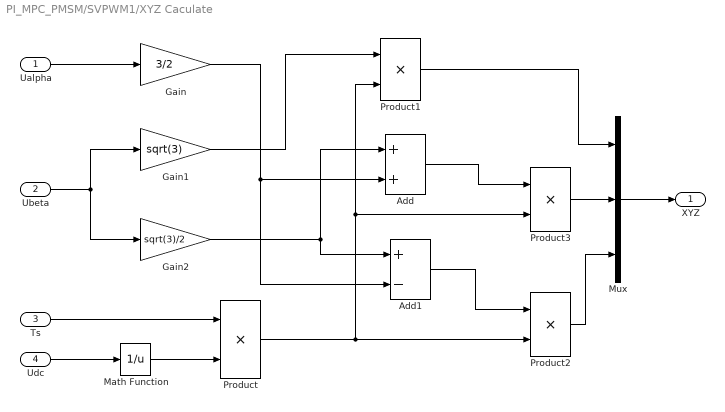
== system PI_MPC_PMSM/SVPWM1/XYZ Caculate ==
  Ualpha : Inport
  Ubeta : Inport  Port=2
  Ts : Inport  Port=3
  Udc : Inport  Port=4
  Add : Sum
  Add1 : Sum  Inputs=+-
  Gain : Gain  Gain=3/2
  Gain1 : Gain  Gain=sqrt(3)
  Gain2 : Gain  Gain=sqrt(3)/2
  Math Function : Math  Operator=reciprocal  SaturateOnIntegerOverflow=on
  Mux : Mux  Inputs=3
  Product{,1..3} (4 alike) : Product  RndMeth=Zero
  XYZ : Outport  VectorParamsAs1DForOutWhenUnconnected=on
  wires:
  Mux/1 -> XYZ/1
  Product1/1 -> Mux/1
  Product3/1 -> Mux/2
  Product2/1 -> Mux/3
  Ualpha/1 -> Gain/1
  Ubeta/1 -> Gain2/1, Gain1/1
  Udc/1 -> Math Function/1
  Math Function/1 -> Product/2
  Ts/1 -> Product/1
  Gain1/1 -> Product1/1
  Product/1 -> Product2/2, Product1/2, Product3/2
  Gain/1 -> Add1/2, Add/2
  Gain2/1 -> Add/1, Add1/1
  Add1/1 -> Product2/1
  Add/1 -> Product3/1

== matlab function PI_MPC_PMSM/电流环MPC控制 ==
  data: uqk input; uq output; uqk1 input; iqk input; iqkm1 input; iqr input
function uq = fcn(uqk,uqk1,iqk,iqkm1,iqr)
% q轴电流的模型预测控制：先基于电机q轴电压方程推导离散化电流预测模型，计算预测时域内仅由历史电流决定的电流预测值及电压对电流的影响系数；
% 通过对比实际预测电流与初步预测电流得到误差，校正电流参考值；
% 最后构建包含电流跟踪误差和控制量变化的目标函数，求解二次规划得到最优电压增量，输出下一时刻q轴电压控制量，实现电流精准跟踪。

% fcn - 永磁同步电机(q轴)电流预测控制核心计算函数
% 输入参数:
%   uqk    : 当前k时刻的q轴电压控制量 (V)
%   uqk1   : 上一时刻(k-1)的q轴电压控制量 (V)
%   iqk    : 当前k时刻的q轴电流反馈值 (A)
%   iqkm1  : 上一时刻(k-1)的q轴电流反馈值 (A)
%   iqr    : q轴电流参考值（电流环给定）(A)
% 输出参数:
%   uq     : 计算得到的下一时刻q轴电压控制量 (V)

%% 1. 定义电机及控制系统固定参数
ff=0.3163;               % 电机相关系数（未在计算中使用）
Rs=0.994;                % 定子相电阻 (Ω)
np=4;                    % 电机极对数（未在计算中使用）
Ts=1e-6;                 % 控制系统采样周期 (s)
Ld=6.3e-3;               % d轴电感 (H)
Lq=9e-3;                 % q轴电感 (H)
delta=0;                 % 误差校正系数（初始化为0，可根据系统调节）
N=4;                     % 模型预测控制(MPC)的预测时域长度
Nu=2;                    % 模型预测控制(MPC)的控制时域长度

%% 2. 推导离散化模型的系数
% 基于电机q轴电压方程：u_q = R_s*i_q + L_q*di_q/dt
% 离散化后得到：i_q(k+1) = C*i_q(k) + D*u_q(k)
C=1-Rs*Ts/Lq;            % 离散化模型系数C
D=Ts/Ld;                 % 离散化模型系数D（注：此处用Ld，需确认是否应为Lq）

%% 3. 初始化数组（存储预测时域内的中间变量）
Wiqm = zeros(N,1);       % 初始化：仅由历史电流决定的q轴电流预测值矩阵
Wuq = zeros(N,1);        % 初始化：电压控制量对电流预测值的影响系数矩阵
Wiqp = zeros(N,1);       % 初始化：综合后的q轴电流预测值矩阵
Iqr  = zeros(N,1);       % 初始化：经误差校正后的q轴电流参考值矩阵

%% 4. 计算预测时域内的电流预测系数矩阵
for i = 1:N
    Ci=0;
    Cj=0;
    Cn=0;
    
    % 计算系数Ci和Cj：用于Wiqm的计算
    for j = 0:N
       Ci = Ci+C^(j);          % 累加计算C的0到N次幂和
       Cj=Ci-1;                % Ci减去1，用于历史电流项的计算
    end
    
    % 计算系数Cn：用于Wuq的计算
    for j = 0:N-1
       Cn = Cn+(N-j)*C^(j);    % 带权重累加C的幂次和，权重为(N-j)
    end
    
    % 计算仅由历史电流决定的电流预测值
    Wiqm(i, 1) = Ci*iqk - Cj*iqkm1;
    % 计算电压控制量对电流预测的影响系数
    Wuq(i, 1) = Cn*D;
end

%% 5. 计算电压增量及初步电流预测值
dtuq0=uqk-uqk1;              % 计算当前时刻与上一时刻的q轴电压增量
Wiqp=Wiqm + Wuq.*dtuq0;      % 结合电压增量，计算初步的q轴电流预测值

%% 6. 误差计算与反馈校正
iqk1=C*iqk + D*uqk;          % 计算k+1时刻的q轴电流实际预测值
e=iqk1 - Wiqp(1,1);          % 计算"初步预测值"与"实际预测值"的误差

% 对预测时域内的电流参考值进行反馈校正（补偿模型误差）
for i = 1:N
    Iqr(i,1) = iqr + delta*e;    % 校正后的电流参考值 = 原始参考值 + 误差补偿项
end

%% 7. 模型预测控制的滚动优化求解
R=0.001*eye(Nu);             % 控制量增量的权重矩阵（惩罚过度的控制量变化）
Q=eye(N);                    % 电流跟踪误差的权重矩阵（强调跟踪精度）

% 求解二次规划问题，最小化目标函数 J = ||Iqr-Wiqm-Wuq*dtuq||_Q^2 + ||dtuq||_R^2
% 解析解：dtuq = inv(R^2 + Wuq'*Q*Wuq) * (Wuq'*Q*(Iqr-Wiqm))
dtuq=inv(R^(2)+Wuq'*Q*Wuq)*(Wuq'*Q*(Iqr-Wiqm));

% 取控制时域第一个控制量，计算最终输出的q轴电压
uq = dtuq(1,1) + uqk1;      % 最终控制量 = 电压增量 + 上一时刻电压值

end

== matlab function PI_MPC_PMSM/转速环MPC控制/MATLAB Function ==
  data: iqk input; iq output; iqk1 input; wk input; wk1 input; wr input; TL input
function iq = fcn(iqk,iqk1,wk,wk1,wr,TL)
% 转速环连续集模型预测控制：基于电机机械运动方程推导转速离散化模型，计算预测时域内仅由历史转速决定的转速预测值及 q 轴电流对转速的影响系数；
% 结合电流增量得到初步转速预测值，对比实际预测转速得到误差并校正转速参考值；
% 通过求解二次规划解析解得到最优q轴电流增量，输出最终q轴电流参考值，实现转速精准跟踪并抑制负载扰动。
%fcn - 永磁同步电机转速环模型预测控制(MPC)核心计算函数
% 输入参数:
%   iqk    : 当前k时刻的q轴电流反馈值 (A)，作为转速环的控制量
%   iqk1   : 上一时刻(k-1)的q轴电流反馈值 (A)
%   wk     : 当前k时刻的电机转速反馈值 (rad/s)
%   wk1    : 上一时刻(k-1)的电机转速反馈值 (rad/s)
%   wr     : 电机转速参考值（转速环给定）(rad/s)
%   TL     : 电机负载转矩扰动 (N·m)
% 输出参数:
%   iq     : 转速环输出的q轴电流参考值（送给电流环）(A)

%% 1. 定义电机及控制系统固定参数
ff=0.3163;               % 电机反电动势系数 (V/(rad/s))
Ts=1e-5;                 % 转速环采样周期 (s)
np=4;                    % 电机极对数
F=0.009;                 % 电机粘滞摩擦系数 (N·m/(rad/s))
J=0.014;                 % 电机转动惯量 (kg·m²)
delta=80;                % 转速预测误差校正系数（调节反馈校正强度）
N=4;                     % 模型预测控制(MPC)的预测时域长度
Nu=2;                    % 模型预测控制(MPC)的控制时域长度

%% 2. 推导转速离散化模型的核心系数
% 基于电机机械运动方程：J*dw/dt = T_e - T_L - F*w
% 电磁转矩 T_e = 1.5*np*ff*iq，代入后离散化得到：w(k+1) = A*w(k) + B*iq(k) - TL*Ts/J
A=1-F*Ts/J;              % 离散化模型系数A（转速自身衰减项）
B=1.5*np*ff*Ts/J;        % 离散化模型系数B（q轴电流对转速的影响项）

%% 3. 初始化数组（存储预测时域内的中间变量）
Wwm = zeros(N,1);        % 初始化：仅由历史转速决定的转速预测值矩阵
Wiq = zeros(N,1);        % 初始化：q轴电流对转速预测值的影响系数矩阵
Wwp = zeros(N,1);        % 初始化：综合后的转速预测值矩阵
Wr  = zeros(N,1);        % 初始化：经误差校正后的转速参考值矩阵
% N=4;  % 重复定义，注释掉（避免变量重复赋值）

%% 4. 计算预测时域内的转速预测系数矩阵
for i = 1:N
    Ai=0;
    Aj=0;
    An=0;
    
    % 计算系数Ai和Aj：用于Wwm（历史转速项）的计算
    for j = 0:N
       Ai = Ai+A^(j);          % 累加计算A的0到N次幂和
       Aj=Ai-1;                % Ai减去1，用于历史转速项的计算
    end
    
    % 计算系数An：用于Wiq（电流影响项）的计算
    for j = 0:N-1
       An = An+(N-j)*A^(j);    % 带权重累加A的幂次和，权重为(N-j)
    end
    
    % 计算仅由历史转速决定的转速预测值
    Wwm(i, 1) = Ai*wk - Aj*wk1;
    % 计算q轴电流对转速预测的影响系数
    Wiq(i, 1) = An*B;
end

%% 5. 计算电流增量及初步转速预测值
dtiq0=iqk-iqk1;              % 计算当前时刻与上一时刻的q轴电流增量
Wwp=Wwm + Wiq.*dtiq0;        % 结合电流增量，计算初步的转速预测值

%% 6. 误差计算与反馈校正（补偿模型误差/扰动）
wmk1=A*wk + B*iqk - TL*Ts/J; % 计算k+1时刻的转速实际预测值（含负载转矩扰动）
e=wmk1 - Wwp(1,1);           % 计算"初步预测值"与"实际预测值"的误差

% 对预测时域内的转速参考值进行反馈校正（补偿模型误差和负载扰动）
for i = 1:N
    Wr(i,1) = wr + delta*e;    % 校正后的转速参考值 = 原始参考值 + 误差补偿项
end

%% 7. 模型预测控制的滚动优化求解
R=eye(Nu);                % 控制量（iq）增量的权重矩阵（惩罚电流突变）
Q=eye(N);                 % 转速跟踪误差的权重矩阵（强调转速跟踪精度）

% 求解二次规划问题，最小化目标函数：J = ||Wr-Wwm-Wiq*dtiq||_Q² + ||dtiq||_R²
% 解析解：dtiq = inv(R² + Wiq'*Q*Wiq) * (Wiq'*Q*(Wr-Wwm))
dtiq=inv(R^(2)+Wiq'*Q*Wiq)*(Wiq'*Q*(Wr-Wwm));

% 取控制时域第一个控制量，计算最终输出的q轴电流参考值
iq = dtiq(1,1) + iqk1;    % 最终iq参考值 = 电流增量 + 上一时刻iq值

end
